simulink model "SeatBeltIndication"  (R2021b)
settings: Solver=FixedStepDiscrete  StartTime=0.0  StopTime=10.0  FixedStep=1  RelTol=1e-3  EnableMultiTasking=on
PreLoadFcn:
  | Ts=1;
settings Model: Creator=adish  LastModifiedBy=adish
settings OptimizationCC: DefaultParameterBehavior=Inlined  UseDivisionForNetSlopeComputation=on  GainParamInheritBuiltInType=on  UseFloatMulNetSlope=on  InlineInvariantSignals=on  EnhancedBackFolding=on  BooleansAsBitfields=on  PassReuseOutputArgsAs=Individual arguments  StateBitsets=on  DataBitsets=on  ZeroExternalMemoryAtStartup=off  ZeroInternalMemoryAtStartup=off  NoFixptDivByZeroProtection=on  EfficientFloat2IntCast=on  LifeSpan=1  OptimizeBlockOrder=speed  DifferentSizesBufferReuse=on  EfficientTunableParamExpr=on
settings DebuggingCC: ParameterTunabilityLossMsg=error
settings HardwareCC: ProdBitPerPointer=32  ProdBitPerSizeT=32  ProdBitPerPtrDiffT=32  ProdLargestAtomicFloat=None  ProdWordSize=32  ProdHWDeviceType=Renesas->RH850
settings SFSimCC: SimGenImportedTypeDefs=on  MATLABDynamicMemAlloc=off
settings RTWCC: Description=AUTOSAR  SystemTargetFile=autosar.tlc  GenCodeOnly=on  PackageGeneratedCodeAndArtifacts=on  PackageName=SeatBeltIndication_autosar_rtw  TemplateMakefile=ert_default_tmf  GenerateReport=on  IncludeHyperlinkInReport=on  LaunchReport=on  GenerateTraceInfo=on  GenerateTraceReportSl=on  GenerateTraceReportSf=on  GenerateWebview=on
settings CodeAppCC: ForceParamTrailComments=on  IgnoreCustomStorageClasses=off  OperatorAnnotations=on  SimulinkDataObjDesc=on  SFDataObjDesc=on  CustomSymbolStrGlobalVar=rt$N$M  CustomSymbolStrType=$N$M  CustomSymbolStrFcn=$N$M$F  CustomSymbolStrMacro=$N$M  InsertBlockDesc=on
settings STFCustomTargetCC: TargetLangStandard=C99 (ISO)  MultiwordLength=256  ParMdlRefBuildCompliant=on  CompOptLevelCompliant=on  IncludeMdlTerminateFcn=off  CombineOutputUpdateFcns=on  CombineSignalStateStructs=on  SuppressErrorStatus=on  ERTCustomFileBanners=on  SupportAbsoluteTime=off  SupportNonFinite=off  SupportComplex=off  SupportContinuousTime=off  SupportNonInlinedSFcns=off  RemoveResetFunc=on  MATLABClassNameForMDSCustomization=Simulink.SoftwareTarget.ERTCustomization  AutosarCompliant=on  GRTInterface=off  UseToolchainInfoCompliant=on  LookupTableObjectStructAxisOrder=2,1,3,4,...  LUTObjectStructOrderEvenSpacing=Size,Table,Breakpoints  SystemTargetFile=autosar.tlc
settings ERTTargetCC: TargetLangStandard=C99 (ISO)  ConcurrentExecutionCompliant=off  IncludeMdlTerminateFcn=off  CombineSignalStateStructs=on  SuppressErrorStatus=on  SupportAbsoluteTime=off  SupportNonFinite=off  SupportComplex=off  ModelStepFunctionPrototypeControlCompliant=off  CPPClassGenCompliant=off  AutosarCompliant=on  LookupTableObjectStructAxisOrder=2,1,3,4,...  LUTObjectStructOrderEvenSpacing=Size,Table,Breakpoints  InlinedParameterPlacement=NonHierarchical  ERTCustomFileTemplate=example_file_process.tlc  ERTFilePackagingFormat=CompactWithDataFile

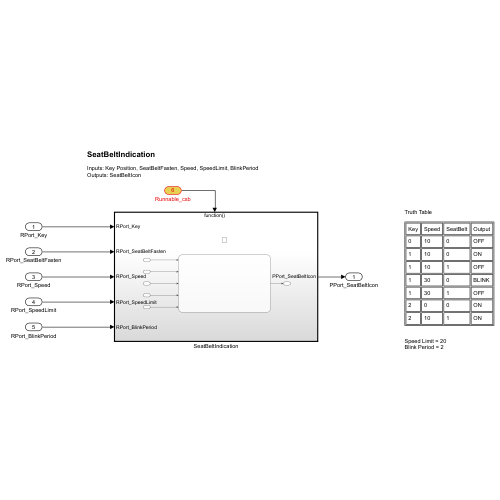
[thumbnail: Simulink's stored preview of the top-level diagram]
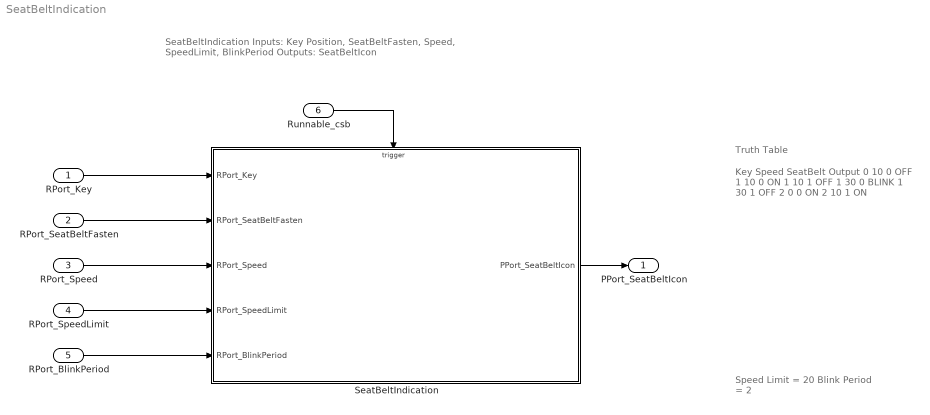
== system SeatBeltIndication ==
  note: Truth Table
  note: Speed Limit = 20
      | Blink Period = 2
  note: Key
      | Speed
      | SeatBelt
      | Output
      |
      | 0
      | 10
      | 0
      | OFF
      |
      | 1
      | 10
      | 0
      | ON
      |
      | 1
      | 10
      | 1
      | OFF
      |
      | 1
      | 30
      | 0
      | BLINK
      |
      | 1
      | 30
      | 1
      | OFF
      |
      | 2
      | 0
      | 0
      | ON
      |
      | 2
      | 10
      | 1
      | ON
  note: SeatBeltIndication
      |
      | Inputs: Key Position, SeatBeltFasten, Speed, SpeedLimit, BlinkPeriod
      | Outputs: SeatBeltIcon
  RPort_Key : Inport
  RPort_SeatBeltFasten : Inport  Port=2
  RPort_Speed : Inport  Port=3
  RPort_SpeedLimit : Inport  Port=4
  RPort_BlinkPeriod : Inport  Port=5
  Runnable_csb : Inport  Port=6  SampleTime=Ts  OutputFunctionCall=on
  SeatBeltIndication : Subsystem  TreatAsAtomicUnit=on
  PPort_SeatBeltIcon : Outport
  wires:
  RPort_Key/1 -> SeatBeltIndication/1(RPort_Key)
  RPort_SeatBeltFasten/1 -> SeatBeltIndication/2(RPort_SeatBeltFasten)
  RPort_Speed/1 -> SeatBeltIndication/3(RPort_Speed)
  RPort_SpeedLimit/1 -> SeatBeltIndication/4(RPort_SpeedLimit)
  RPort_BlinkPeriod/1 -> SeatBeltIndication/5(RPort_BlinkPeriod)
  SeatBeltIndication/1(PPort_SeatBeltIcon) -> PPort_SeatBeltIcon/1
  Runnable_csb/1 -> SeatBeltIndication/Trigger

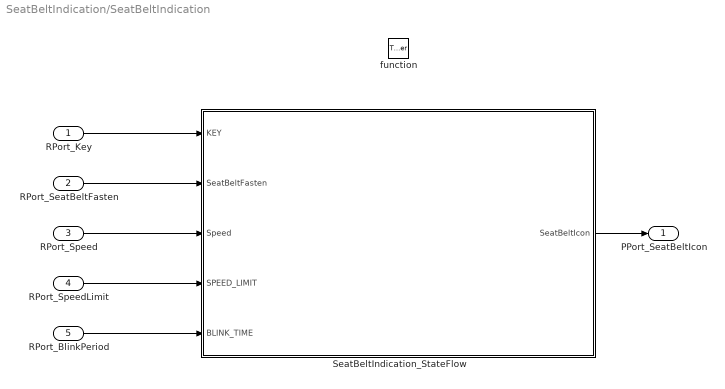
== system SeatBeltIndication/SeatBeltIndication ==
  RPort_Key : Inport
  RPort_SeatBeltFasten : Inport  Port=2
  RPort_Speed : Inport  Port=3
  RPort_SpeedLimit : Inport  Port=4
  RPort_BlinkPeriod : Inport  Port=5
  function : TriggerPort  TriggerType=function-call  VariantControl=(inherit)  SampleTimeType=periodic  SampleTime=-1
  SeatBeltIndication_StateFlow : Stateflow chart  TreatAsAtomicUnit=on
  PPort_SeatBeltIcon : Outport
  wires:
  RPort_SeatBeltFasten/1 -> SeatBeltIndication_StateFlow/2(SeatBeltFasten)
  RPort_BlinkPeriod/1 -> SeatBeltIndication_StateFlow/5(BLINK_TIME)
  RPort_SpeedLimit/1 -> SeatBeltIndication_StateFlow/4(SPEED_LIMIT)
  RPort_Speed/1 -> SeatBeltIndication_StateFlow/3(Speed)
  RPort_Key/1 -> SeatBeltIndication_StateFlow/1(KEY)
  SeatBeltIndication_StateFlow/1(SeatBeltIcon) -> PPort_SeatBeltIcon/1

== stateflow chart SeatBeltIndication/SeatBeltIndication_StateFlow ==
  state KEY_OFF
    entry: SeatBeltIcon=0;
  state KEY_CRANK
    entry: SeatBeltIcon=1;
  state KEY_ON
    state SB_UNFASTEN
      state LOW_SPEED
        entry: SeatBeltIcon = 1;
      state HIGH_SPEED
        state OFF
          entry: SeatBeltIcon=0;
        state ON
          entry: SeatBeltIcon=1;
        (default) -> OFF
        ON -> OFF : [after(BLINK_TIME,sec)]
        OFF -> ON : [after(BLINK_TIME,sec)]
      (default) -> LOW_SPEED
      LOW_SPEED -> HIGH_SPEED : [Speed > SPEED_LIMIT]
      HIGH_SPEED -> LOW_SPEED : [Speed <= SPEED_LIMIT]
    state SB_FASTEN
      en: SeatBeltIcon=0;
    (default) -> (junction 12)
    (junction 12) -> SB_UNFASTEN [order 2]
    (junction 12) -> SB_FASTEN [order 1] : [SeatBeltFasten == 1]
    SB_UNFASTEN -> SB_FASTEN : [SeatBeltFasten == 1]
    SB_FASTEN -> SB_UNFASTEN : [SeatBeltFasten == 0]
  (default) -> KEY_OFF
  KEY_OFF -> KEY_ON : [KEY==1]
  KEY_ON -> KEY_OFF [order 1] : [KEY == 0]
  KEY_ON -> KEY_CRANK [order 2] : [KEY == 2]
  KEY_CRANK -> KEY_ON : [KEY == 1]
  data: KEY input; SeatBeltFasten input; Speed input; SeatBeltIcon output; SPEED_LIMIT input; BLINK_TIME input
